simulink library "CAN_Lib_V1"  (R2018b)
settings: Solver=VariableStepAuto  StartTime=0.0  StopTime=10.0  RelTol=1e-3
undefined symbols (not defined in the file): canChannel
libraries: canmsglib x158, canlib x35, simulink x1
(part 1 of 11)
settings Model: ModifiedHistory=CAN Bus model library  Creator=E00026  LastModifiedBy=E00026
settings DataIOCC: ReturnWorkspaceOutputs=on

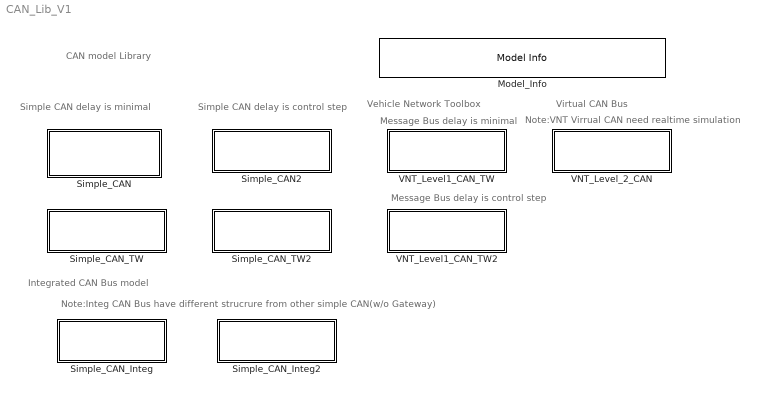
== system CAN_Lib_V1 ==
  note: Note:VNT Virrual CAN need realtime simulation
  note: Note:Integ CAN Bus have different strucrure from other simple CAN(w/o Gateway)
  note: Integrated CAN Bus model
  note: Virtual CAN Bus
  note: Message Bus delay is minimal
  note: Simple CAN delay is minimal
  note: CAN model Library
  note: Vehicle Network Toolbox
  note: Simple CAN delay is control step
  note: Message Bus delay is control step
  Model_Info : simulink/Model-Wide Utilities/Model Info  Frame=on  DisplayStringWithTags=|  HorizontalTextAlignment=Left  LeftAlignmentValue=0.02
      | Version  %<ModelVersion>
      | LastModifided by %<LastModifiedBy>  Date %<LastModificationDate>
      | Description  %<Description>
  Simple_CAN : Subsystem  VariantControl=VarObj_CanType_Simpl
  Simple_CAN2 : Subsystem  VariantControl=VarObj_CanType_Simpl
  Simple_CAN_Integ : Subsystem  VariantControl=VarObj_CanType_Simpl
  Simple_CAN_Integ2 : Subsystem  VariantControl=VarObj_CanType_Simpl
  Simple_CAN_TW : Subsystem  VariantControl=VarObj_CanType_Simpl_TW
  Simple_CAN_TW2 : Subsystem  VariantControl=VarObj_CanType_Simpl_TW
  VNT_Level1_CAN_TW : Subsystem  VariantControl=VarObj_CanType_VNT_Level_1
  VNT_Level1_CAN_TW2 : Subsystem  VariantControl=VarObj_CanType_Simpl_TW
  VNT_Level_2_CAN : Subsystem  VariantControl=VarObj_CanType_VNT_simu

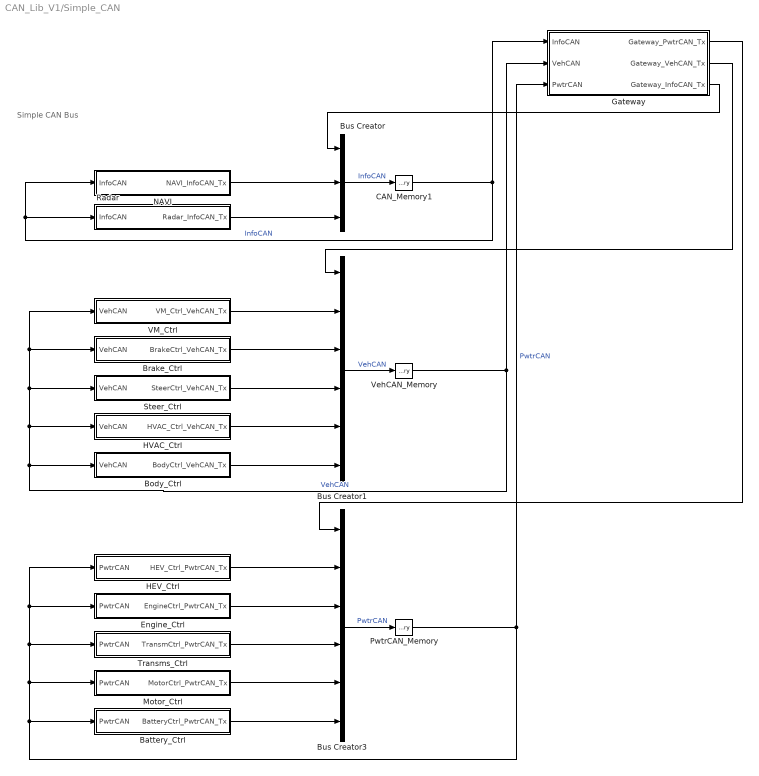
== system CAN_Lib_V1/Simple_CAN ==
  note: Simple CAN Bus
  Battery_Ctrl : Subsystem
  Body_Ctrl : Subsystem
  Brake_Ctrl : Subsystem
  Bus Creator : BusCreator  Inputs=3
  Bus Creator1 : BusCreator  Inputs=6
  Bus Creator3 : BusCreator  Inputs=6
  CAN_Memory1 : Memory
  Engine_Ctrl : Subsystem
  Gateway : Subsystem
  HEV_Ctrl : Subsystem
  HVAC_Ctrl : Subsystem
  Motor_Ctrl : Subsystem
  NAVI : Subsystem
  PwtrCAN_Memory : Memory
  Radar : Subsystem
  Steer_Ctrl : Subsystem
  Transms_Ctrl : Subsystem
  VM_Ctrl : Subsystem
  VehCAN_Memory : Memory
  wires:
  Bus Creator3/1 -> PwtrCAN_Memory/1  "PwtrCAN"
  HEV_Ctrl/1(HEV_Ctrl_PwtrCAN_Tx) -> Bus Creator3/2
  Bus Creator/1 -> CAN_Memory1/1  "InfoCAN"
  PwtrCAN_Memory/1 -> Motor_Ctrl/1(PwtrCAN), Transms_Ctrl/1(PwtrCAN), Engine_Ctrl/1(PwtrCAN), HEV_Ctrl/1(PwtrCAN), Battery_Ctrl/1(PwtrCAN), Gateway/3(PwtrCAN)  "PwtrCAN"
  Engine_Ctrl/1(EngineCtrl_PwtrCAN_Tx) -> Bus Creator3/3
  Transms_Ctrl/1(TransmCtrl_PwtrCAN_Tx) -> Bus Creator3/4
  Bus Creator1/1 -> VehCAN_Memory/1  "VehCAN"
  Battery_Ctrl/1(BatteryCtrl_PwtrCAN_Tx) -> Bus Creator3/6
  Body_Ctrl/1(BodyCtrl_VehCAN_Tx) -> Bus Creator1/6
  VehCAN_Memory/1 -> Gateway/2(VehCAN), HVAC_Ctrl/1(VehCAN), Brake_Ctrl/1(VehCAN), VM_Ctrl/1(VehCAN), Steer_Ctrl/1(VehCAN), Body_Ctrl/1(VehCAN)  "VehCAN"
  VM_Ctrl/1(VM_Ctrl_VehCAN_Tx) -> Bus Creator1/2
  Radar/1(Radar_InfoCAN_Tx) -> Bus Creator/3
  NAVI/1(NAVI_InfoCAN_Tx) -> Bus Creator/2
  Steer_Ctrl/1(SteerCtrl_VehCAN_Tx) -> Bus Creator1/4
  HVAC_Ctrl/1(HVAC_Ctrl_VehCAN_Tx) -> Bus Creator1/5
  Motor_Ctrl/1(MotorCtrl_PwtrCAN_Tx) -> Bus Creator3/5
  Brake_Ctrl/1(BrakeCtrl_VehCAN_Tx) -> Bus Creator1/3
  CAN_Memory1/1 -> Gateway/1(InfoCAN), NAVI/1(InfoCAN), Radar/1(InfoCAN)  "InfoCAN"
  Gateway/3(Gateway_InfoCAN_Tx) -> Bus Creator/1
  Gateway/2(Gateway_VehCAN_Tx) -> Bus Creator1/1
  Gateway/1(Gateway_PwtrCAN_Tx) -> Bus Creator3/1

== system CAN_Lib_V1/Simple_CAN2 ==
  note: Simple CAN Bus
  Battery_Ctrl : Subsystem
  Body_Ctrl : Subsystem
  Brake_Ctrl : Subsystem
  Bus Creator : BusCreator  Inputs=3
  Bus Creator1 : BusCreator  Inputs=6
  Bus Creator3 : BusCreator  Inputs=6
  Engine_Ctrl : Subsystem
  Gateway : Subsystem
  HEV_Ctrl : Subsystem
  HVAC_Ctrl : Subsystem
  Motor_Ctrl : Subsystem
  NAVI : Subsystem
  Radar : Subsystem
  Steer_Ctrl : Subsystem
  Transms_Ctrl : Subsystem
  VM_Ctrl : Subsystem
  wires:
  Gateway/1(Gateway_PwtrCAN_Tx) -> Bus Creator3/1
  Gateway/2(Gateway_VehCAN_Tx) -> Bus Creator1/1
  Gateway/3(Gateway_InfoCAN_Tx) -> Bus Creator/1
  Brake_Ctrl/1(BrakeCtrl_VehCAN_Tx) -> Bus Creator1/3
  Motor_Ctrl/1(MotorCtrl_PwtrCAN_Tx) -> Bus Creator3/5
  HVAC_Ctrl/1(HVAC_Ctrl_VehCAN_Tx) -> Bus Creator1/5
  Steer_Ctrl/1(SteerCtrl_VehCAN_Tx) -> Bus Creator1/4
  NAVI/1(NAVI_InfoCAN_Tx) -> Bus Creator/2
  Radar/1(Radar_InfoCAN_Tx) -> Bus Creator/3
  VM_Ctrl/1(VM_Ctrl_VehCAN_Tx) -> Bus Creator1/2
  Body_Ctrl/1(BodyCtrl_VehCAN_Tx) -> Bus Creator1/6
  Battery_Ctrl/1(BatteryCtrl_PwtrCAN_Tx) -> Bus Creator3/6
  Bus Creator1/1 -> Body_Ctrl/1(VehCAN), Steer_Ctrl/1(VehCAN), VM_Ctrl/1(VehCAN), Brake_Ctrl/1(VehCAN), HVAC_Ctrl/1(VehCAN), Gateway/2(VehCAN)  "VehCAN"
  Transms_Ctrl/1(TransmCtrl_PwtrCAN_Tx) -> Bus Creator3/4
  Engine_Ctrl/1(EngineCtrl_PwtrCAN_Tx) -> Bus Creator3/3
  Bus Creator/1 -> Radar/1(InfoCAN), NAVI/1(InfoCAN), Gateway/1(InfoCAN)  "InfoCAN"
  HEV_Ctrl/1(HEV_Ctrl_PwtrCAN_Tx) -> Bus Creator3/2
  Bus Creator3/1 -> Gateway/3(PwtrCAN), Battery_Ctrl/1(PwtrCAN), HEV_Ctrl/1(PwtrCAN), Engine_Ctrl/1(PwtrCAN), Transms_Ctrl/1(PwtrCAN), Motor_Ctrl/1(PwtrCAN)  "PwtrCAN"

== system CAN_Lib_V1/Simple_CAN_Integ ==
  note: Simple CAN Integrated Bus
  Battery_Ctrl : Subsystem
  Body_Ctrl : Subsystem
  Brake_Ctrl : Subsystem
  Bus Creator : BusCreator  Inputs=2
  Bus Creator1 : BusCreator  Inputs=5
  Bus Creator2 : BusCreator  Inputs=3
  Bus Creator3 : BusCreator  Inputs=5
  Engine_Ctrl : Subsystem
  HEV_Ctrl : Subsystem
  HVAC_Ctrl : Subsystem
  IntegCAN_Memory : Memory
  Motor_Ctrl : Subsystem
  NAVI : Subsystem
  Radar : Subsystem
  Steer_Ctrl : Subsystem
  Transms_Ctrl : Subsystem
  VM_Ctrl : Subsystem
  tag scope: CAN=scoped
  wires:
  Bus Creator2/1 -> IntegCAN_Memory/1
  IntegCAN_Memory/1 -> Battery_Ctrl/1(CAN), Motor_Ctrl/1(CAN), Transms_Ctrl/1(CAN), Engine_Ctrl/1(CAN), HEV_Ctrl/1(CAN), Body_Ctrl/1(CAN), HVAC_Ctrl/1(CAN), Steer_Ctrl/1(CAN), VM_Ctrl/1(CAN), Radar/1(CAN), NAVI/1(CAN), Brake_Ctrl/1(CAN), [CAN]  "CAN"
  Brake_Ctrl/1(BrakeCtrl_VehCAN_Tx) -> Bus Creator1/2
  Motor_Ctrl/1(MotorCtrl_PwtrCAN_Tx) -> Bus Creator3/4
  HVAC_Ctrl/1(HVAC_Ctrl_VehCAN_Tx) -> Bus Creator1/4
  Steer_Ctrl/1(SteerCtrl_VehCAN_Tx) -> Bus Creator1/3
  NAVI/1(NAVI_InfoCAN_Tx) -> Bus Creator/1
  Radar/1(Radar_InfoCAN_Tx) -> Bus Creator/2
  VM_Ctrl/1(VM_Ctrl_VehCAN_Tx) -> Bus Creator1/1
  Body_Ctrl/1(BodyCtrl_VehCAN_Tx) -> Bus Creator1/5
  Battery_Ctrl/1(BatteryCtrl_PwtrCAN_Tx) -> Bus Creator3/5
  Bus Creator1/1 -> Bus Creator2/2  "VehCAN"
  Transms_Ctrl/1(TransmCtrl_PwtrCAN_Tx) -> Bus Creator3/3
  Engine_Ctrl/1(EngineCtrl_PwtrCAN_Tx) -> Bus Creator3/2
  Bus Creator/1 -> Bus Creator2/1  "InfoCAN"
  HEV_Ctrl/1(HEV_Ctrl_PwtrCAN_Tx) -> Bus Creator3/1
  Bus Creator3/1 -> Bus Creator2/3  "PwtrCAN"

== system CAN_Lib_V1/Simple_CAN_Integ2 ==
  note: Simple CAN Integrated Bus
  Battery_Ctrl : Subsystem
  Body_Ctrl : Subsystem
  Brake_Ctrl : Subsystem
  Bus Creator : BusCreator  Inputs=2
  Bus Creator1 : BusCreator  Inputs=5
  Bus Creator2 : BusCreator  Inputs=3
  Bus Creator3 : BusCreator  Inputs=5
  Engine_Ctrl : Subsystem
  HEV_Ctrl : Subsystem
  HVAC_Ctrl : Subsystem
  Motor_Ctrl : Subsystem
  NAVI : Subsystem
  Radar : Subsystem
  Steer_Ctrl : Subsystem
  Transms_Ctrl : Subsystem
  VM_Ctrl : Subsystem
  tag scope: CAN=scoped
  wires:
  Bus Creator2/1 -> Battery_Ctrl/1(CAN), Motor_Ctrl/1(CAN), Transms_Ctrl/1(CAN), Engine_Ctrl/1(CAN), HEV_Ctrl/1(CAN), Body_Ctrl/1(CAN), HVAC_Ctrl/1(CAN), Steer_Ctrl/1(CAN), VM_Ctrl/1(CAN), Radar/1(CAN), NAVI/1(CAN), Brake_Ctrl/1(CAN), [CAN]  "CAN"
  Brake_Ctrl/1(BrakeCtrl_VehCAN_Tx) -> Bus Creator1/2
  Motor_Ctrl/1(MotorCtrl_PwtrCAN_Tx) -> Bus Creator3/4
  HVAC_Ctrl/1(HVAC_Ctrl_VehCAN_Tx) -> Bus Creator1/4
  Steer_Ctrl/1(SteerCtrl_VehCAN_Tx) -> Bus Creator1/3
  NAVI/1(NAVI_InfoCAN_Tx) -> Bus Creator/1
  Radar/1(Radar_InfoCAN_Tx) -> Bus Creator/2
  VM_Ctrl/1(VM_Ctrl_VehCAN_Tx) -> Bus Creator1/1
  Body_Ctrl/1(BodyCtrl_VehCAN_Tx) -> Bus Creator1/5
  Battery_Ctrl/1(BatteryCtrl_PwtrCAN_Tx) -> Bus Creator3/5
  Bus Creator1/1 -> Bus Creator2/2  "VehCAN"
  Transms_Ctrl/1(TransmCtrl_PwtrCAN_Tx) -> Bus Creator3/3
  Engine_Ctrl/1(EngineCtrl_PwtrCAN_Tx) -> Bus Creator3/2
  Bus Creator/1 -> Bus Creator2/1  "InfoCAN"
  HEV_Ctrl/1(HEV_Ctrl_PwtrCAN_Tx) -> Bus Creator3/1
  Bus Creator3/1 -> Bus Creator2/3  "PwtrCAN"

== system CAN_Lib_V1/Simple_CAN_TW ==
  note: Simple CAN Bus
  Battery_Ctrl : Subsystem
  Body_Ctrl : Subsystem
  Brake_Ctrl : Subsystem
  Engine_Ctrl : Subsystem
  Gateway : Subsystem
  HEV_Ctrl : Subsystem
  HVAC_Ctrl : Subsystem
  InfoCAN : Subsystem
  Motor_Ctrl : Subsystem
  NAVI : Subsystem
  PwtrCAN : Subsystem
  Radar : Subsystem
  Steer_Ctrl : Subsystem
  Transms_Ctrl : Subsystem
  VM_Ctrl : Subsystem
  VehCAN : Subsystem
  connections:
  InfoCAN/LConn1 -- NAVI/RConn1
  InfoCAN/LConn2 -- Radar/RConn1
  Gateway/LConn1 -- InfoCAN/RConn1
  VehCAN/RConn1 -- Gateway/LConn2
  Gateway/RConn1 -- PwtrCAN/LConn1
  VM_Ctrl/RConn1 -- VehCAN/LConn1
  Brake_Ctrl/RConn1 -- VehCAN/LConn2
  Steer_Ctrl/RConn1 -- VehCAN/LConn3
  HVAC_Ctrl/RConn1 -- VehCAN/LConn4
  Body_Ctrl/RConn1 -- VehCAN/LConn5
  PwtrCAN/RConn1 -- HEV_Ctrl/LConn1
  PwtrCAN/RConn2 -- Engine_Ctrl/LConn1
  PwtrCAN/RConn3 -- Transms_Ctrl/LConn1
  PwtrCAN/RConn4 -- Motor_Ctrl/LConn1
  PwtrCAN/RConn5 -- Battery_Ctrl/LConn1

== system CAN_Lib_V1/Simple_CAN_TW2 ==
  note: Simple CAN Bus
  Battery_Ctrl : Subsystem
  Body_Ctrl : Subsystem
  Brake_Ctrl : Subsystem
  Engine_Ctrl : Subsystem
  Gateway : Subsystem
  HEV_Ctrl : Subsystem
  HVAC_Ctrl : Subsystem
  InfoCAN : Subsystem
  Motor_Ctrl : Subsystem
  NAVI : Subsystem
  PwtrCAN : Subsystem
  Radar : Subsystem
  Steer_Ctrl : Subsystem
  Transms_Ctrl : Subsystem
  VM_Ctrl : Subsystem
  VehCAN : Subsystem
  connections:
  PwtrCAN/RConn5 -- Battery_Ctrl/LConn1
  PwtrCAN/RConn4 -- Motor_Ctrl/LConn1
  PwtrCAN/RConn3 -- Transms_Ctrl/LConn1
  PwtrCAN/RConn2 -- Engine_Ctrl/LConn1
  PwtrCAN/RConn1 -- HEV_Ctrl/LConn1
  Body_Ctrl/RConn1 -- VehCAN/LConn5
  HVAC_Ctrl/RConn1 -- VehCAN/LConn4
  Steer_Ctrl/RConn1 -- VehCAN/LConn3
  Brake_Ctrl/RConn1 -- VehCAN/LConn2
  VM_Ctrl/RConn1 -- VehCAN/LConn1
  Gateway/RConn1 -- PwtrCAN/LConn1
  VehCAN/RConn1 -- Gateway/LConn2
  Gateway/LConn1 -- InfoCAN/RConn1
  InfoCAN/LConn2 -- Radar/RConn1
  InfoCAN/LConn1 -- NAVI/RConn1

== system CAN_Lib_V1/VNT_Level1_CAN_TW ==
  note: VNT Level1 CAN Bus
  Battery_Ctrl : Subsystem
  Body_Ctrl : Subsystem
  Brake_Ctrl : Subsystem
  Engine_Ctrl : Subsystem
  Gateway : Subsystem
  HEV_Ctrl : Subsystem
  HVAC_Ctrl : Subsystem
  InfoCAN : Subsystem
  Motor_Ctrl : Subsystem
  NAVI : Subsystem
  PwtrCAN : Subsystem
  Radar : Subsystem
  Steer_Ctrl : Subsystem
  Transms_Ctrl : Subsystem
  VM_Ctrl : Subsystem
  VehCAN : Subsystem
  connections:
  InfoCAN/LConn1 -- NAVI/RConn1
  InfoCAN/LConn2 -- Radar/RConn1
  Gateway/LConn1 -- InfoCAN/RConn1
  VehCAN/RConn1 -- Gateway/LConn2
  Gateway/RConn1 -- PwtrCAN/LConn1
  VM_Ctrl/RConn1 -- VehCAN/LConn1
  Brake_Ctrl/RConn1 -- VehCAN/LConn2
  Steer_Ctrl/RConn1 -- VehCAN/LConn3
  HVAC_Ctrl/RConn1 -- VehCAN/LConn4
  Body_Ctrl/RConn1 -- VehCAN/LConn5
  PwtrCAN/RConn1 -- HEV_Ctrl/LConn1
  PwtrCAN/RConn2 -- Engine_Ctrl/LConn1
  PwtrCAN/RConn3 -- Transms_Ctrl/LConn1
  PwtrCAN/RConn4 -- Motor_Ctrl/LConn1
  PwtrCAN/RConn5 -- Battery_Ctrl/LConn1

== system CAN_Lib_V1/VNT_Level1_CAN_TW2 ==
  note: VNT Level1 CAN Bus
  Battery_Ctrl : Subsystem
  Body_Ctrl : Subsystem
  Brake_Ctrl : Subsystem
  Engine_Ctrl : Subsystem
  Gateway : Subsystem
  HEV_Ctrl : Subsystem
  HVAC_Ctrl : Subsystem
  InfoCAN : Subsystem
  Motor_Ctrl : Subsystem
  NAVI : Subsystem
  PwtrCAN : Subsystem
  Radar : Subsystem
  Steer_Ctrl : Subsystem
  Transms_Ctrl : Subsystem
  VM_Ctrl : Subsystem
  VehCAN : Subsystem
  connections:
  PwtrCAN/RConn5 -- Battery_Ctrl/LConn1
  PwtrCAN/RConn4 -- Motor_Ctrl/LConn1
  PwtrCAN/RConn3 -- Transms_Ctrl/LConn1
  PwtrCAN/RConn2 -- Engine_Ctrl/LConn1
  PwtrCAN/RConn1 -- HEV_Ctrl/LConn1
  Body_Ctrl/RConn1 -- VehCAN/LConn5
  HVAC_Ctrl/RConn1 -- VehCAN/LConn4
  Steer_Ctrl/RConn1 -- VehCAN/LConn3
  Brake_Ctrl/RConn1 -- VehCAN/LConn2
  VM_Ctrl/RConn1 -- VehCAN/LConn1
  Gateway/RConn1 -- PwtrCAN/LConn1
  VehCAN/RConn1 -- Gateway/LConn2
  Gateway/LConn1 -- InfoCAN/RConn1
  InfoCAN/LConn2 -- Radar/RConn1
  InfoCAN/LConn1 -- NAVI/RConn1

== system CAN_Lib_V1/VNT_Level_2_CAN ==
  note: VNT Level_2 CAN Bus
  Battery_Ctrl : Subsystem
  Body_Ctrl : Subsystem
  Brake_Ctrl : Subsystem
  CAN Configuration : canlib/CAN Configuration  BlockHandle=36204.0016  DeviceMenu=MathWorks Virtual 1 (Channel 1)  Device=MathWorks Virtual 1 (Channel 1)  ObjConstructor=canChannel('MathWorks','Virtual 1',1)  BusSpeed=500000  EnableBitParameters=off  AckMode=Normal
      settings: SourceProductName=Vehicle Network Toolbox  SourceProductBaseCode=VN
  CAN Configuration1 : canlib/CAN Configuration  BlockHandle=36205.0016  DeviceMenu=MathWorks Virtual 1 (Channel 2)  Device=MathWorks Virtual 1 (Channel 2)  ObjConstructor=canChannel('MathWorks','Virtual 1',2)  BusSpeed=500000  EnableBitParameters=off  AckMode=Normal
      settings: SourceProductName=Vehicle Network Toolbox  SourceProductBaseCode=VN
  Engine_Ctrl : Subsystem
  Gateway : Subsystem
  HEV_Ctrl : Subsystem
  HVAC_Ctrl : Subsystem
  Motor_Ctrl : Subsystem
  NAVI : Subsystem
  Radar : Subsystem
  Steer_Ctrl : Subsystem
  Transms_Ctrl : Subsystem
  VM_Ctrl : Subsystem

== system CAN_Lib_V1/Simple_CAN/Battery_Ctrl ==
  note: Battery control
  note: CAN receive and transmit
  note: Battery Control
  PwtrCAN : Inport
  Bus Creator5 : BusCreator  Inputs=1
  Bus Selector : BusSelector  OutputSignals=HEV_Ctrl_PwtrCAN_Tx.HEVCtrl_Motor_torque_request
  Rate Transition1 : RateTransition  Deterministic=off
      settings: AttributesFormatString=<Deterministic=%<Deterministic>>
  Rate Transition2 : RateTransition  Deterministic=off
      settings: AttributesFormatString=<Deterministic=%<Deterministic>>
  BatteryCtrl_PwtrCAN_Tx : Outport
  tag scope: BatteryCtrl_PwtrCAN_Rx=scoped
  wires:
  Bus Selector/1 -> Bus Creator5/1  "<HEVCtrl_Motor_torque_request>"
  PwtrCAN/1 -> Bus Selector/1
  Bus Creator5/1 -> Rate Transition1/1
  [BatteryCtrl_PwtrCAN_Tx] -> Rate Transition2/1
  Rate Transition1/1 -> [BatteryCtrl_PwtrCAN_Rx]  "BatteryCtrl_PwtrCAN_Rx"
  Rate Transition2/1 -> BatteryCtrl_PwtrCAN_Tx/1  "BatteryCtrl_PwtrCAN_Tx"

== system CAN_Lib_V1/Simple_CAN/Body_Ctrl ==
  note: Body control
  note: CAN receive and transmit
  note: Body Control
  VehCAN : Inport
  Bus Creator : BusCreator  Inputs=3
  Bus Selector3 : BusSelector  OutputSignals=BrakeCtrl_VehCAN_Tx.BrkCtrl_Vehicle_speed,Gateway_VehCAN_Tx.EngCtrl_Engine_speed,Gateway_VehCAN_Tx.HEVCtrl_IdleStop_status
  Rate Transition1 : RateTransition  Deterministic=off
      settings: AttributesFormatString=<Deterministic=%<Deterministic>>
  Rate Transition2 : RateTransition  Deterministic=off
      settings: AttributesFormatString=<Deterministic=%<Deterministic>>
  BodyCtrl_VehCAN_Tx : Outport
  tag scope: BodyCtrl_VehCAN_Rx=scoped
  wires:
  Bus Creator/1 -> Rate Transition1/1
  Bus Selector3/1 -> Bus Creator/1  "<BrkCtrl_Vehicle_speed>"
  Bus Selector3/2 -> Bus Creator/2  "<EngCtrl_Engine_speed>"
  VehCAN/1 -> Bus Selector3/1
  [BodyCtrl_VehCAN_Tx] -> Rate Transition2/1
  Rate Transition1/1 -> [BodyCtrl_VehCAN_Rx]  "BodyCtrl_VehCAN_Rx"
  Rate Transition2/1 -> BodyCtrl_VehCAN_Tx/1  "BodyCtrl_VehCAN_Tx"
  Bus Selector3/3 -> Bus Creator/3  "<HEVCtrl_IdleStop_status>"

== system CAN_Lib_V1/Simple_CAN/Brake_Ctrl ==
  note: Brake control
  note: CAN receive and transmit
  note: Brake Control
  VehCAN : Inport
  Bus Creator : BusCreator  Inputs=4
  Bus Selector3 : BusSelector  OutputSignals=Gateway_VehCAN_Tx.HEVCtrl_Regen_brake_torque_available,Gateway_VehCAN_Tx.HEVCtrl_Regen_brake_torque_actual,VM_Ctrl_VehCAN_Tx.VMCtrl_BrakeForceStatus,VM_Ctrl_VehCAN_Tx.VMCtrl_BrakeForceCmnd
  Rate Transition1 : RateTransition  Deterministic=off
      settings: AttributesFormatString=<Deterministic=%<Deterministic>>
  Rate Transition2 : RateTransition  Deterministic=off
      settings: AttributesFormatString=<Deterministic=%<Deterministic>>
  BrakeCtrl_VehCAN_Tx : Outport
  tag scope: BrakeCtrl_VehCAN_Rx=scoped
  wires:
  Bus Creator/1 -> Rate Transition1/1
  Bus Selector3/2 -> Bus Creator/2  "<HEVCtrl_Regen_brake_torque_actual>"
  Bus Selector3/1 -> Bus Creator/1  "<HEVCtrl_Regen_brake_torque_available>"
  VehCAN/1 -> Bus Selector3/1
  [BrakeCtrl_VehCAN_Tx] -> Rate Transition2/1
  Rate Transition1/1 -> [BrakeCtrl_VehCAN_Rx]  "BrakeCtrl_VehCAN_Rx"
  Rate Transition2/1 -> BrakeCtrl_VehCAN_Tx/1  "BrakeCtrl_VehCAN_Tx"
  Bus Selector3/3 -> Bus Creator/3  "<VMCtrl_BrakeForceStatus>"
  Bus Selector3/4 -> Bus Creator/4  "<VMCtrl_BrakeForceCmnd>"

== system CAN_Lib_V1/Simple_CAN/Engine_Ctrl ==
  note: Engine control
  note: Engine Control
  note: CAN receive and transmit
  PwtrCAN : Inport
  Bus Creator5 : BusCreator  Inputs=4
  Bus Selector : BusSelector  OutputSignals=HEV_Ctrl_PwtrCAN_Tx.HEVCtrl_Engine_torque_request,HEV_Ctrl_PwtrCAN_Tx.HEVCtrl_IdleStop_preparation_request,HEV_Ctrl_PwtrCAN_Tx.HEVCtrl_IdleStop_request,HEV_Ctrl_PwtrCAN_Tx.HEVCtrl_IdleStop_status
  Rate Transition1 : RateTransition  Deterministic=off
      settings: AttributesFormatString=<Deterministic=%<Deterministic>>
  Rate Transition2 : RateTransition  Deterministic=off
      settings: AttributesFormatString=<Deterministic=%<Deterministic>>
  EngineCtrl_PwtrCAN_Tx : Outport
  tag scope: EngineCtrl_PwtrCAN_Rx=scoped
  wires:
  [EngineCtrl_PwtrCAN_Tx] -> Rate Transition2/1
  PwtrCAN/1 -> Bus Selector/1
  Bus Creator5/1 -> Rate Transition1/1
  Bus Selector/1 -> Bus Creator5/1  "<HEVCtrl_Engine_torque_request>"
  Rate Transition1/1 -> [EngineCtrl_PwtrCAN_Rx]  "EngineCtrl_PwtrCAN_Rx"
  Rate Transition2/1 -> EngineCtrl_PwtrCAN_Tx/1  "EngineCtrl_PwtrCAN_Tx"
  Bus Selector/2 -> Bus Creator5/2  "<HEVCtrl_IdleStop_preparation_request>"
  Bus Selector/3 -> Bus Creator5/3  "<HEVCtrl_IdleStop_request>"
  Bus Selector/4 -> Bus Creator5/4  "<HEVCtrl_IdleStop_status>"

== system CAN_Lib_V1/Simple_CAN/Gateway ==
  note: Gateway
  InfoCAN : Inport
  VehCAN : Inport  Port=2
  PwtrCAN : Inport  Port=3
  Gateway_InfoCAN : Subsystem
  Gateway_PwtrCAN : Subsystem
  Gateway_VehCAN : Subsystem
  Info Hub : Subsystem
  Gateway_PwtrCAN_Tx : Outport
  Gateway_VehCAN_Tx : Outport  Port=2
  Gateway_InfoCAN_Tx : Outport  Port=3
  wires:
  InfoCAN/1 -> Info Hub/1(InfoCAN), Gateway_PwtrCAN/1(InfoCAN), Gateway_VehCAN/1(InfoCAN)
  PwtrCAN/1 -> Info Hub/3(PwtrCAN), Gateway_VehCAN/2(PwtrCAN)
  VehCAN/1 -> Gateway_InfoCAN/1(VehCAN), Info Hub/2(VehCAN), Gateway_PwtrCAN/2(VehCAN)
  Gateway_InfoCAN/1(Gateway_InfoCAN_Tx) -> Gateway_InfoCAN_Tx/1
  Gateway_VehCAN/1(Gateway_VehCAN_Tx) -> Gateway_VehCAN_Tx/1
  Gateway_PwtrCAN/1(Gateway_PwtrCAN_Tx) -> Gateway_PwtrCAN_Tx/1

== system CAN_Lib_V1/Simple_CAN/HEV_Ctrl ==
  note: HEV control
  note: HEV control
  note: CAN receive and transmit
  PwtrCAN : Inport
  Bus Creator1 : BusCreator  Inputs=13
  Bus Selector3 : BusSelector  OutputSignals=BatteryCtrl_PwtrCAN_Tx.BatCtrl_SOC,TransmCtrl_PwtrCAN_Tx.TmCtrl_Clutch_position,TransmCtrl_PwtrCAN_Tx.TmCtrl_Gear_position,Gateway_PwtrCAN_Tx.BrkCtrl_Vehicle_speed,Gateway_PwtrCAN_Tx.BrkCtrl_Regen_brake_torque_request,MotorCtrl_PwtrCAN_Tx.MtrCtrl_Motor_torque_actual,MotorCtrl_PwtrCAN_Tx.MtrCtrl_Motor_torque_available,MotorCtrl_PwtrCAN_Tx.MtrCtrl_Motor_regen_torque_available,EngineCtrl_PwtrCAN_Tx.EngCtrl_Engine_speed,EngineCtrl_PwtrCAN_Tx.EngCtrl_Engine_torque_actual,Gateway_PwtrCAN_Tx.VMCtrl_PropTorqStatus,Gateway_PwtrCAN_Tx.VMCtrl_PropTorqCmnd,Gateway_PwtrCAN_Tx.NAVI_Home_around_status
  Rate Transition1 : RateTransition  Deterministic=off
      settings: AttributesFormatString=<Deterministic=%<Deterministic>>
  Rate Transition4 : RateTransition  Deterministic=off
      settings: AttributesFormatString=<Deterministic=%<Deterministic>>
  HEV_Ctrl_PwtrCAN_Tx : Outport
  tag scope: HEV_Ctrl_PwtrCAN_Rx=scoped
  wires:
  Bus Creator1/1 -> Rate Transition1/1
  Bus Selector3/10 -> Bus Creator1/10  "<EngCtrl_Engine_torque_actual>"
  Bus Selector3/9 -> Bus Creator1/9  "<EngCtrl_Engine_speed>"
  Bus Selector3/8 -> Bus Creator1/8  "<MtrCtrl_Motor_regen_torque_available>"
  Bus Selector3/7 -> Bus Creator1/7  "<MtrCtrl_Motor_torque_available>"
  Bus Selector3/6 -> Bus Creator1/6  "<MtrCtrl_Motor_torque_actual>"
  Bus Selector3/5 -> Bus Creator1/5  "<BrkCtrl_Regen_brake_torque_request>"
  Bus Selector3/4 -> Bus Creator1/4  "<BrkCtrl_Vehicle_speed>"
  Bus Selector3/3 -> Bus Creator1/3  "<TmCtrl_Gear_position>"
  Bus Selector3/2 -> Bus Creator1/2  "<TmCtrl_Clutch_position>"
  Bus Selector3/1 -> Bus Creator1/1  "<BatCtrl_SOC>"
  PwtrCAN/1 -> Bus Selector3/1
  [HEV_Ctrl_PwtrCAN_Tx] -> Rate Transition4/1
  Rate Transition4/1 -> HEV_Ctrl_PwtrCAN_Tx/1  "HEV_Ctrl_PwtrCAN_Tx"
  Rate Transition1/1 -> [HEV_Ctrl_PwtrCAN_Rx]  "HEV_Ctrl_PwtrCAN_Rx"
  Bus Selector3/11 -> Bus Creator1/11  "<VMCtrl_PropTorqStatus>"
  Bus Selector3/12 -> Bus Creator1/12  "<VMCtrl_PropTorqCmnd>"
  Bus Selector3/13 -> Bus Creator1/13  "<NAVI_Home_around_status>"

== system CAN_Lib_V1/Simple_CAN/HVAC_Ctrl ==
  note: HVAC control
  note: CAN receive and transmit
  note: HVAC Control
  VehCAN : Inport
  Bus Creator : BusCreator  Inputs=3
  Bus Selector : BusSelector  OutputSignals=Gateway_VehCAN_Tx.EngCtrl_Engine_speed,Gateway_VehCAN_Tx.HEVCtrl_IdleStop_preparation_request,Gateway_VehCAN_Tx.HEVCtrl_IdleStop_status
  Rate Transition1 : RateTransition  Deterministic=off
      settings: AttributesFormatString=<Deterministic=%<Deterministic>>
  Rate Transition2 : RateTransition  Deterministic=off
      settings: AttributesFormatString=<Deterministic=%<Deterministic>>
  HVAC_Ctrl_VehCAN_Tx : Outport
  tag scope: HVAC_Ctrl_VehCAN_Rx=scoped
  wires:
  Bus Creator/1 -> Rate Transition1/1
  Bus Selector/1 -> Bus Creator/1  "<EngCtrl_Engine_speed>"
  VehCAN/1 -> Bus Selector/1
  [HVAC_Ctrl_VehCAN_Tx] -> Rate Transition2/1
  Rate Transition1/1 -> [HVAC_Ctrl_VehCAN_Rx]  "HVAC_Ctrl_VehCAN_Rx"
  Rate Transition2/1 -> HVAC_Ctrl_VehCAN_Tx/1  "HVAC_Ctrl_VehCAN_Tx"
  Bus Selector/2 -> Bus Creator/2  "<HEVCtrl_IdleStop_preparation_request>"
  Bus Selector/3 -> Bus Creator/3  "<HEVCtrl_IdleStop_status>"

== system CAN_Lib_V1/Simple_CAN/Motor_Ctrl ==
  note: Motor control
  note: Motor Control
  note: CAN receive and transmit
  PwtrCAN : Inport
  Bus Creator7 : BusCreator  Inputs=3
  Bus Selector2 : BusSelector  OutputSignals=TransmCtrl_PwtrCAN_Tx.TmCtrl_Clutch_position,HEV_Ctrl_PwtrCAN_Tx.HEVCtrl_Motor_torque_request,EngineCtrl_PwtrCAN_Tx.EngCtrl_Engine_speed
  Rate Transition1 : RateTransition  Deterministic=off
      settings: AttributesFormatString=<Deterministic=%<Deterministic>>
  Rate Transition2 : RateTransition  Deterministic=off
      settings: AttributesFormatString=<Deterministic=%<Deterministic>>
  MotorCtrl_PwtrCAN_Tx : Outport
  tag scope: MotorCtrl_PwtrCAN_Rx=scoped
  wires:
  [MotorCtrl_PwtrCAN_Tx] -> Rate Transition2/1
  Rate Transition1/1 -> [MotorCtrl_PwtrCAN_Rx]  "MotorCtrl_PwtrCAN_Rx"
  Bus Selector2/2 -> Bus Creator7/2  "<HEVCtrl_Motor_torque_request>"
  Bus Creator7/1 -> Rate Transition1/1
  Bus Selector2/3 -> Bus Creator7/3  "<EngCtrl_Engine_speed>"
  Bus Selector2/1 -> Bus Creator7/1  "<TmCtrl_Clutch_position>"
  Rate Transition2/1 -> MotorCtrl_PwtrCAN_Tx/1  "MotorCtrl_PwtrCAN_Tx"
  PwtrCAN/1 -> Bus Selector2/1

== system CAN_Lib_V1/Simple_CAN/NAVI ==
  note: Navigation
  note: CAN receive and transmit
  note: Navigation
  InfoCAN : Inport
  Bus Creator : BusCreator  Inputs=1
  Bus Selector1 : BusSelector  OutputSignals=Gateway_InfoCAN_Tx.BrkCtrl_Vehicle_speed
  Rate Transition1 : RateTransition  Deterministic=off
      settings: AttributesFormatString=<Deterministic=%<Deterministic>>
  Rate Transition2 : RateTransition  Deterministic=off
      settings: AttributesFormatString=<Deterministic=%<Deterministic>>
  NAVI_InfoCAN_Tx : Outport
  tag scope: NAVI_InfoCAN_Rx=scoped
  wires:
  Bus Creator/1 -> Rate Transition1/1
  Bus Selector1/1 -> Bus Creator/1  "<BrkCtrl_Vehicle_speed>"
  InfoCAN/1 -> Bus Selector1/1
  [NAVI_InfoCAN_Tx] -> Rate Transition2/1
  Rate Transition1/1 -> [NAVI_InfoCAN_Rx]  "NAVI_InfoCAN_Rx"
  Rate Transition2/1 -> NAVI_InfoCAN_Tx/1  "NAVI_InfoCAN_Tx"

== system CAN_Lib_V1/Simple_CAN/Radar ==
  note: Radar detection
  note: CAN receive and transmit
  note: Radar Detection
  InfoCAN : Inport
  Bus Creator : BusCreator  Inputs=1
  Bus Selector1 : BusSelector  OutputSignals=Gateway_InfoCAN_Tx.BrkCtrl_Vehicle_speed
  Rate Transition1 : RateTransition  Deterministic=off
      settings: AttributesFormatString=<Deterministic=%<Deterministic>>
  Rate Transition2 : RateTransition  Deterministic=off
      settings: AttributesFormatString=<Deterministic=%<Deterministic>>
  Radar_InfoCAN_Tx : Outport
  tag scope: Radar_InfoCAN_Rx=scoped
  wires:
  InfoCAN/1 -> Bus Selector1/1
  Bus Creator/1 -> Rate Transition1/1
  Bus Selector1/1 -> Bus Creator/1  "<BrkCtrl_Vehicle_speed>"
  [Radar_InfoCAN_Tx] -> Rate Transition2/1
  Rate Transition1/1 -> [Radar_InfoCAN_Rx]  "Radar_InfoCAN_Rx"
  Rate Transition2/1 -> Radar_InfoCAN_Tx/1  "Radar_InfoCAN_Tx"

== system CAN_Lib_V1/Simple_CAN/Steer_Ctrl ==
  note: Steering control
  note: CAN receive and transmit
  note: Steering Control
  VehCAN : Inport
  Bus Creator : BusCreator  Inputs=1
  Bus Selector1 : BusSelector  OutputSignals=BrakeCtrl_VehCAN_Tx.BrkCtrl_Vehicle_speed
  Rate Transition1 : RateTransition  Deterministic=off
      settings: AttributesFormatString=<Deterministic=%<Deterministic>>
  Rate Transition2 : RateTransition  Deterministic=off
      settings: AttributesFormatString=<Deterministic=%<Deterministic>>
  SteerCtrl_VehCAN_Tx : Outport
  tag scope: SteerCtrl_VehCAN_Rx=scoped
  wires:
  Bus Creator/1 -> Rate Transition1/1
  Bus Selector1/1 -> Bus Creator/1  "<BrkCtrl_Vehicle_speed>"
  VehCAN/1 -> Bus Selector1/1
  [SteerCtrl_VehCAN_Tx] -> Rate Transition2/1
  Rate Transition1/1 -> [SteerCtrl_VehCAN_Rx]  "SteerCtrl_VehCAN_Rx"
  Rate Transition2/1 -> SteerCtrl_VehCAN_Tx/1  "SteerCtrl_VehCAN_Tx"

== system CAN_Lib_V1/Simple_CAN/Transms_Ctrl ==
  note: Transmission control
  note: CAN receive and transmit
  note: Transmission Control
  PwtrCAN : Inport
  Bus Creator6 : BusCreator  Inputs=2
  Bus Selector1 : BusSelector  OutputSignals=Gateway_PwtrCAN_Tx.BrkCtrl_Vehicle_speed,EngineCtrl_PwtrCAN_Tx.EngCtrl_Engine_speed
  Rate Transition1 : RateTransition  Deterministic=off
      settings: AttributesFormatString=<Deterministic=%<Deterministic>>
  Rate Transition2 : RateTransition  Deterministic=off
      settings: AttributesFormatString=<Deterministic=%<Deterministic>>
  TransmCtrl_PwtrCAN_Tx : Outport
  tag scope: TransmCtrl_PwtrCAN_Rx=scoped
  wires:
  [TransmCtrl_PwtrCAN_Tx] -> Rate Transition2/1
  Rate Transition2/1 -> TransmCtrl_PwtrCAN_Tx/1  "TransmCtrl_PwtrCAN_Tx"
  Bus Creator6/1 -> Rate Transition1/1
  Bus Selector1/2 -> Bus Creator6/2  "<EngCtrl_Engine_speed>"
  Bus Selector1/1 -> Bus Creator6/1  "<BrkCtrl_Vehicle_speed>"
  PwtrCAN/1 -> Bus Selector1/1
  Rate Transition1/1 -> [TransmCtrl_PwtrCAN_Rx]  "TransmCtrl_PwtrCAN_Rx"

== system CAN_Lib_V1/Simple_CAN/VM_Ctrl ==
  note: Vehicle motion control
  note: Vehicle Motion Control
  note: CAN receive and transmit
  VehCAN : Inport
  Bus Creator : BusCreator  Inputs=1
  Bus Selector1 : BusSelector  OutputSignals=BrakeCtrl_VehCAN_Tx.BrkCtrl_Vehicle_speed
  Rate Transition1 : RateTransition  Deterministic=off
      settings: AttributesFormatString=<Deterministic=%<Deterministic>>
  Rate Transition2 : RateTransition  Deterministic=off
      settings: AttributesFormatString=<Deterministic=%<Deterministic>>
  VM_Ctrl_VehCAN_Tx : Outport
  tag scope: VM_Ctrl_VehCAN_Rx=scoped
  wires:
  Bus Creator/1 -> Rate Transition1/1
  Bus Selector1/1 -> Bus Creator/1  "<BrkCtrl_Vehicle_speed>"
  VehCAN/1 -> Bus Selector1/1
  [VM_Ctrl_VehCAN_Tx] -> Rate Transition2/1
  Rate Transition1/1 -> [VM_Ctrl_VehCAN_Rx]  "VM_Ctrl_VehCAN_Rx"
  Rate Transition2/1 -> VM_Ctrl_VehCAN_Tx/1  "VM_Ctrl_VehCAN_Tx"

== system CAN_Lib_V1/Simple_CAN2/Battery_Ctrl ==
  note: Battery Control
  note: CAN receive and transmit
  note: Battery control
  PwtrCAN : Inport
  Bus Creator5 : BusCreator  Inputs=1
  Bus Selector : BusSelector  OutputSignals=HEV_Ctrl_PwtrCAN_Tx.HEVCtrl_Motor_torque_request
  Rate Transition1 : RateTransition  Deterministic=off
      settings: AttributesFormatString=<Deterministic=%<Deterministic>>
  Unit Delay : UnitDelay  SampleTime=-1
  BatteryCtrl_PwtrCAN_Tx : Outport
  tag scope: BatteryCtrl_PwtrCAN_Rx=scoped
  wires:
  Unit Delay/1 -> BatteryCtrl_PwtrCAN_Tx/1  "BatteryCtrl_PwtrCAN_Tx"
  Rate Transition1/1 -> [BatteryCtrl_PwtrCAN_Rx]  "BatteryCtrl_PwtrCAN_Rx"
  [BatteryCtrl_PwtrCAN_Tx] -> Unit Delay/1
  Bus Creator5/1 -> Rate Transition1/1
  PwtrCAN/1 -> Bus Selector/1
  Bus Selector/1 -> Bus Creator5/1  "<HEVCtrl_Motor_torque_request>"

== system CAN_Lib_V1/Simple_CAN2/Body_Ctrl ==
  note: Body Control
  note: CAN receive and transmit
  note: Body control
  VehCAN : Inport
  Bus Creator : BusCreator  Inputs=3
  Bus Selector3 : BusSelector  OutputSignals=BrakeCtrl_VehCAN_Tx.BrkCtrl_Vehicle_speed,Gateway_VehCAN_Tx.EngCtrl_Engine_speed,Gateway_VehCAN_Tx.HEVCtrl_IdleStop_status
  Rate Transition1 : RateTransition  Deterministic=off
      settings: AttributesFormatString=<Deterministic=%<Deterministic>>
  Unit Delay : UnitDelay  SampleTime=-1
  BodyCtrl_VehCAN_Tx : Outport
  tag scope: BodyCtrl_VehCAN_Rx=scoped
  wires:
  Bus Selector3/3 -> Bus Creator/3  "<HEVCtrl_IdleStop_status>"
  Unit Delay/1 -> BodyCtrl_VehCAN_Tx/1  "BodyCtrl_VehCAN_Tx"
  Rate Transition1/1 -> [BodyCtrl_VehCAN_Rx]  "BodyCtrl_VehCAN_Rx"
  [BodyCtrl_VehCAN_Tx] -> Unit Delay/1
  VehCAN/1 -> Bus Selector3/1
  Bus Selector3/2 -> Bus Creator/2  "<EngCtrl_Engine_speed>"
  Bus Selector3/1 -> Bus Creator/1  "<BrkCtrl_Vehicle_speed>"
  Bus Creator/1 -> Rate Transition1/1

== system CAN_Lib_V1/Simple_CAN2/Brake_Ctrl ==
  note: Brake Control
  note: CAN receive and transmit
  note: Brake control
  VehCAN : Inport
  Bus Creator : BusCreator  Inputs=4
  Bus Selector3 : BusSelector  OutputSignals=Gateway_VehCAN_Tx.HEVCtrl_Regen_brake_torque_available,Gateway_VehCAN_Tx.HEVCtrl_Regen_brake_torque_actual,VM_Ctrl_VehCAN_Tx.VMCtrl_BrakeForceStatus,VM_Ctrl_VehCAN_Tx.VMCtrl_BrakeForceCmnd
  Rate Transition1 : RateTransition  Deterministic=off
      settings: AttributesFormatString=<Deterministic=%<Deterministic>>
  Unit Delay : UnitDelay  SampleTime=-1
  BrakeCtrl_VehCAN_Tx : Outport
  tag scope: BrakeCtrl_VehCAN_Rx=scoped
  wires:
  Bus Selector3/4 -> Bus Creator/4  "<VMCtrl_BrakeForceCmnd>"
  Bus Selector3/3 -> Bus Creator/3  "<VMCtrl_BrakeForceStatus>"
  Unit Delay/1 -> BrakeCtrl_VehCAN_Tx/1  "BrakeCtrl_VehCAN_Tx"
  Rate Transition1/1 -> [BrakeCtrl_VehCAN_Rx]  "BrakeCtrl_VehCAN_Rx"
  [BrakeCtrl_VehCAN_Tx] -> Unit Delay/1
  VehCAN/1 -> Bus Selector3/1
  Bus Selector3/1 -> Bus Creator/1  "<HEVCtrl_Regen_brake_torque_available>"
  Bus Selector3/2 -> Bus Creator/2  "<HEVCtrl_Regen_brake_torque_actual>"
  Bus Creator/1 -> Rate Transition1/1

== system CAN_Lib_V1/Simple_CAN2/Engine_Ctrl ==
  note: CAN receive and transmit
  note: Engine Control
  note: Engine control
  PwtrCAN : Inport
  Bus Creator5 : BusCreator  Inputs=4
  Bus Selector : BusSelector  OutputSignals=HEV_Ctrl_PwtrCAN_Tx.HEVCtrl_Engine_torque_request,HEV_Ctrl_PwtrCAN_Tx.HEVCtrl_IdleStop_preparation_request,HEV_Ctrl_PwtrCAN_Tx.HEVCtrl_IdleStop_request,HEV_Ctrl_PwtrCAN_Tx.HEVCtrl_IdleStop_status
  Rate Transition1 : RateTransition  Deterministic=off
      settings: AttributesFormatString=<Deterministic=%<Deterministic>>
  Unit Delay : UnitDelay  SampleTime=-1
  EngineCtrl_PwtrCAN_Tx : Outport
  tag scope: EngineCtrl_PwtrCAN_Rx=scoped
  wires:
  Bus Selector/4 -> Bus Creator5/4  "<HEVCtrl_IdleStop_status>"
  Bus Selector/3 -> Bus Creator5/3  "<HEVCtrl_IdleStop_request>"
  Bus Selector/2 -> Bus Creator5/2  "<HEVCtrl_IdleStop_preparation_request>"
  Unit Delay/1 -> EngineCtrl_PwtrCAN_Tx/1  "EngineCtrl_PwtrCAN_Tx"
  Rate Transition1/1 -> [EngineCtrl_PwtrCAN_Rx]  "EngineCtrl_PwtrCAN_Rx"
  Bus Selector/1 -> Bus Creator5/1  "<HEVCtrl_Engine_torque_request>"
  Bus Creator5/1 -> Rate Transition1/1
  PwtrCAN/1 -> Bus Selector/1
  [EngineCtrl_PwtrCAN_Tx] -> Unit Delay/1

== system CAN_Lib_V1/Simple_CAN2/Gateway ==
  note: Gateway
  InfoCAN : Inport
  VehCAN : Inport  Port=2
  PwtrCAN : Inport  Port=3
  Gateway_InfoCAN : Subsystem
  Gateway_PwtrCAN : Subsystem
  Gateway_VehCAN : Subsystem
  Info Hub : Subsystem
  Gateway_PwtrCAN_Tx : Outport
  Gateway_VehCAN_Tx : Outport  Port=2
  Gateway_InfoCAN_Tx : Outport  Port=3
  wires:
  Gateway_PwtrCAN/1(Gateway_PwtrCAN_Tx) -> Gateway_PwtrCAN_Tx/1
  Gateway_VehCAN/1(Gateway_VehCAN_Tx) -> Gateway_VehCAN_Tx/1
  Gateway_InfoCAN/1(Gateway_InfoCAN_Tx) -> Gateway_InfoCAN_Tx/1
  VehCAN/1 -> Gateway_PwtrCAN/2(VehCAN), Info Hub/2(VehCAN), Gateway_InfoCAN/1(VehCAN)
  PwtrCAN/1 -> Gateway_VehCAN/2(PwtrCAN), Info Hub/3(PwtrCAN)
  InfoCAN/1 -> Gateway_VehCAN/1(InfoCAN), Gateway_PwtrCAN/1(InfoCAN), Info Hub/1(InfoCAN)

== system CAN_Lib_V1/Simple_CAN2/HEV_Ctrl ==
  note: CAN receive and transmit
  note: HEV control
  note: HEV control
  PwtrCAN : Inport
  Bus Creator1 : BusCreator  Inputs=13
  Bus Selector3 : BusSelector  OutputSignals=BatteryCtrl_PwtrCAN_Tx.BatCtrl_SOC,TransmCtrl_PwtrCAN_Tx.TmCtrl_Clutch_position,TransmCtrl_PwtrCAN_Tx.TmCtrl_Gear_position,Gateway_PwtrCAN_Tx.BrkCtrl_Vehicle_speed,Gateway_PwtrCAN_Tx.BrkCtrl_Regen_brake_torque_request,MotorCtrl_PwtrCAN_Tx.MtrCtrl_Motor_torque_actual,MotorCtrl_PwtrCAN_Tx.MtrCtrl_Motor_torque_available,MotorCtrl_PwtrCAN_Tx.MtrCtrl_Motor_regen_torque_available,EngineCtrl_PwtrCAN_Tx.EngCtrl_Engine_speed,EngineCtrl_PwtrCAN_Tx.EngCtrl_Engine_torque_actual,Gateway_PwtrCAN_Tx.VMCtrl_PropTorqStatus,Gateway_PwtrCAN_Tx.VMCtrl_PropTorqCmnd,Gateway_PwtrCAN_Tx.NAVI_Home_around_status
  Rate Transition1 : RateTransition  Deterministic=off
      settings: AttributesFormatString=<Deterministic=%<Deterministic>>
  Unit Delay : UnitDelay  SampleTime=-1
  HEV_Ctrl_PwtrCAN_Tx : Outport
  tag scope: HEV_Ctrl_PwtrCAN_Rx=scoped
  wires:
  Bus Selector3/13 -> Bus Creator1/13  "<NAVI_Home_around_status>"
  Bus Selector3/12 -> Bus Creator1/12  "<VMCtrl_PropTorqCmnd>"
  Bus Selector3/11 -> Bus Creator1/11  "<VMCtrl_PropTorqStatus>"
  Rate Transition1/1 -> [HEV_Ctrl_PwtrCAN_Rx]  "HEV_Ctrl_PwtrCAN_Rx"
  Unit Delay/1 -> HEV_Ctrl_PwtrCAN_Tx/1  "HEV_Ctrl_PwtrCAN_Tx"
  [HEV_Ctrl_PwtrCAN_Tx] -> Unit Delay/1
  PwtrCAN/1 -> Bus Selector3/1
  Bus Selector3/1 -> Bus Creator1/1  "<BatCtrl_SOC>"
  Bus Selector3/2 -> Bus Creator1/2  "<TmCtrl_Clutch_position>"
  Bus Selector3/3 -> Bus Creator1/3  "<TmCtrl_Gear_position>"
  Bus Selector3/4 -> Bus Creator1/4  "<BrkCtrl_Vehicle_speed>"
  Bus Selector3/5 -> Bus Creator1/5  "<BrkCtrl_Regen_brake_torque_request>"
  Bus Selector3/6 -> Bus Creator1/6  "<MtrCtrl_Motor_torque_actual>"
  Bus Selector3/7 -> Bus Creator1/7  "<MtrCtrl_Motor_torque_available>"
  Bus Selector3/8 -> Bus Creator1/8  "<MtrCtrl_Motor_regen_torque_available>"
  Bus Selector3/9 -> Bus Creator1/9  "<EngCtrl_Engine_speed>"
  Bus Selector3/10 -> Bus Creator1/10  "<EngCtrl_Engine_torque_actual>"
  Bus Creator1/1 -> Rate Transition1/1

== system CAN_Lib_V1/Simple_CAN2/HVAC_Ctrl ==
  note: HVAC Control
  note: CAN receive and transmit
  note: HVAC control
  VehCAN : Inport
  Bus Creator : BusCreator  Inputs=3
  Bus Selector : BusSelector  OutputSignals=Gateway_VehCAN_Tx.EngCtrl_Engine_speed,Gateway_VehCAN_Tx.HEVCtrl_IdleStop_preparation_request,Gateway_VehCAN_Tx.HEVCtrl_IdleStop_status
  Rate Transition1 : RateTransition  Deterministic=off
      settings: AttributesFormatString=<Deterministic=%<Deterministic>>
  Unit Delay : UnitDelay  SampleTime=-1
  HVAC_Ctrl_VehCAN_Tx : Outport
  tag scope: HVAC_Ctrl_VehCAN_Rx=scoped
  wires:
  Bus Selector/3 -> Bus Creator/3  "<HEVCtrl_IdleStop_status>"
  Bus Selector/2 -> Bus Creator/2  "<HEVCtrl_IdleStop_preparation_request>"
  Unit Delay/1 -> HVAC_Ctrl_VehCAN_Tx/1  "HVAC_Ctrl_VehCAN_Tx"
  Rate Transition1/1 -> [HVAC_Ctrl_VehCAN_Rx]  "HVAC_Ctrl_VehCAN_Rx"
  [HVAC_Ctrl_VehCAN_Tx] -> Unit Delay/1
  VehCAN/1 -> Bus Selector/1
  Bus Selector/1 -> Bus Creator/1  "<EngCtrl_Engine_speed>"
  Bus Creator/1 -> Rate Transition1/1

== system CAN_Lib_V1/Simple_CAN2/Motor_Ctrl ==
  note: CAN receive and transmit
  note: Motor Control
  note: Motor control
  PwtrCAN : Inport
  Bus Creator7 : BusCreator  Inputs=3
  Bus Selector2 : BusSelector  OutputSignals=TransmCtrl_PwtrCAN_Tx.TmCtrl_Clutch_position,HEV_Ctrl_PwtrCAN_Tx.HEVCtrl_Motor_torque_request,EngineCtrl_PwtrCAN_Tx.EngCtrl_Engine_speed
  Rate Transition1 : RateTransition  Deterministic=off
      settings: AttributesFormatString=<Deterministic=%<Deterministic>>
  Unit Delay : UnitDelay  SampleTime=-1
  MotorCtrl_PwtrCAN_Tx : Outport
  tag scope: MotorCtrl_PwtrCAN_Rx=scoped
  wires:
  PwtrCAN/1 -> Bus Selector2/1
  Unit Delay/1 -> MotorCtrl_PwtrCAN_Tx/1  "MotorCtrl_PwtrCAN_Tx"
  Bus Selector2/1 -> Bus Creator7/1  "<TmCtrl_Clutch_position>"
  Bus Selector2/3 -> Bus Creator7/3  "<EngCtrl_Engine_speed>"
  Bus Creator7/1 -> Rate Transition1/1
  Bus Selector2/2 -> Bus Creator7/2  "<HEVCtrl_Motor_torque_request>"
  Rate Transition1/1 -> [MotorCtrl_PwtrCAN_Rx]  "MotorCtrl_PwtrCAN_Rx"
  [MotorCtrl_PwtrCAN_Tx] -> Unit Delay/1

== system CAN_Lib_V1/Simple_CAN2/NAVI ==
  note: Navigation
  note: CAN receive and transmit
  note: Navigation
  InfoCAN : Inport
  Bus Creator : BusCreator  Inputs=1
  Bus Selector1 : BusSelector  OutputSignals=Gateway_InfoCAN_Tx.BrkCtrl_Vehicle_speed
  Rate Transition1 : RateTransition  Deterministic=off
      settings: AttributesFormatString=<Deterministic=%<Deterministic>>
  Unit Delay : UnitDelay  SampleTime=-1
  NAVI_InfoCAN_Tx : Outport
  tag scope: NAVI_InfoCAN_Rx=scoped
  wires:
  Unit Delay/1 -> NAVI_InfoCAN_Tx/1  "NAVI_InfoCAN_Tx"
  Rate Transition1/1 -> [NAVI_InfoCAN_Rx]  "NAVI_InfoCAN_Rx"
  [NAVI_InfoCAN_Tx] -> Unit Delay/1
  InfoCAN/1 -> Bus Selector1/1
  Bus Selector1/1 -> Bus Creator/1  "<BrkCtrl_Vehicle_speed>"
  Bus Creator/1 -> Rate Transition1/1

== system CAN_Lib_V1/Simple_CAN2/Radar ==
  note: Radar Detection
  note: CAN receive and transmit
  note: Radar detection
  InfoCAN : Inport
  Bus Creator : BusCreator  Inputs=1
  Bus Selector1 : BusSelector  OutputSignals=Gateway_InfoCAN_Tx.BrkCtrl_Vehicle_speed
  Rate Transition1 : RateTransition  Deterministic=off
      settings: AttributesFormatString=<Deterministic=%<Deterministic>>
  Unit Delay : UnitDelay  SampleTime=-1
  Radar_InfoCAN_Tx : Outport
  tag scope: Radar_InfoCAN_Rx=scoped
  wires:
  Unit Delay/1 -> Radar_InfoCAN_Tx/1  "Radar_InfoCAN_Tx"
  Rate Transition1/1 -> [Radar_InfoCAN_Rx]  "Radar_InfoCAN_Rx"
  [Radar_InfoCAN_Tx] -> Unit Delay/1
  Bus Selector1/1 -> Bus Creator/1  "<BrkCtrl_Vehicle_speed>"
  Bus Creator/1 -> Rate Transition1/1
  InfoCAN/1 -> Bus Selector1/1

== system CAN_Lib_V1/Simple_CAN2/Steer_Ctrl ==
  note: Steering Control
  note: CAN receive and transmit
  note: Steering control
  VehCAN : Inport
  Bus Creator : BusCreator  Inputs=1
  Bus Selector1 : BusSelector  OutputSignals=BrakeCtrl_VehCAN_Tx.BrkCtrl_Vehicle_speed
  Rate Transition1 : RateTransition  Deterministic=off
      settings: AttributesFormatString=<Deterministic=%<Deterministic>>
  Unit Delay : UnitDelay  SampleTime=-1
  SteerCtrl_VehCAN_Tx : Outport
  tag scope: SteerCtrl_VehCAN_Rx=scoped
  wires:
  Unit Delay/1 -> SteerCtrl_VehCAN_Tx/1  "SteerCtrl_VehCAN_Tx"
  Rate Transition1/1 -> [SteerCtrl_VehCAN_Rx]  "SteerCtrl_VehCAN_Rx"
  [SteerCtrl_VehCAN_Tx] -> Unit Delay/1
  VehCAN/1 -> Bus Selector1/1
  Bus Selector1/1 -> Bus Creator/1  "<BrkCtrl_Vehicle_speed>"
  Bus Creator/1 -> Rate Transition1/1

== system CAN_Lib_V1/Simple_CAN2/Transms_Ctrl ==
  note: Transmission Control
  note: CAN receive and transmit
  note: Transmission control
  PwtrCAN : Inport
  Bus Creator6 : BusCreator  Inputs=2
  Bus Selector1 : BusSelector  OutputSignals=Gateway_PwtrCAN_Tx.BrkCtrl_Vehicle_speed,EngineCtrl_PwtrCAN_Tx.EngCtrl_Engine_speed
  Rate Transition1 : RateTransition  Deterministic=off
      settings: AttributesFormatString=<Deterministic=%<Deterministic>>
  Unit Delay : UnitDelay  SampleTime=-1
  TransmCtrl_PwtrCAN_Tx : Outport
  tag scope: TransmCtrl_PwtrCAN_Rx=scoped
  wires:
  Rate Transition1/1 -> [TransmCtrl_PwtrCAN_Rx]  "TransmCtrl_PwtrCAN_Rx"
  PwtrCAN/1 -> Bus Selector1/1
  Bus Selector1/1 -> Bus Creator6/1  "<BrkCtrl_Vehicle_speed>"
  Bus Selector1/2 -> Bus Creator6/2  "<EngCtrl_Engine_speed>"
  Bus Creator6/1 -> Rate Transition1/1
  Unit Delay/1 -> TransmCtrl_PwtrCAN_Tx/1  "TransmCtrl_PwtrCAN_Tx"
  [TransmCtrl_PwtrCAN_Tx] -> Unit Delay/1

== system CAN_Lib_V1/Simple_CAN2/VM_Ctrl ==
  note: CAN receive and transmit
  note: Vehicle Motion Control
  note: Vehicle motion control
  VehCAN : Inport
  Bus Creator : BusCreator  Inputs=1
  Bus Selector1 : BusSelector  OutputSignals=BrakeCtrl_VehCAN_Tx.BrkCtrl_Vehicle_speed
  Rate Transition1 : RateTransition  Deterministic=off
      settings: AttributesFormatString=<Deterministic=%<Deterministic>>
  Unit Delay : UnitDelay  SampleTime=-1
  VM_Ctrl_VehCAN_Tx : Outport
  tag scope: VM_Ctrl_VehCAN_Rx=scoped
  wires:
  Unit Delay/1 -> VM_Ctrl_VehCAN_Tx/1  "VM_Ctrl_VehCAN_Tx"
  Rate Transition1/1 -> [VM_Ctrl_VehCAN_Rx]  "VM_Ctrl_VehCAN_Rx"
  [VM_Ctrl_VehCAN_Tx] -> Unit Delay/1
  VehCAN/1 -> Bus Selector1/1
  Bus Selector1/1 -> Bus Creator/1  "<BrkCtrl_Vehicle_speed>"
  Bus Creator/1 -> Rate Transition1/1

== system CAN_Lib_V1/Simple_CAN_Integ/Battery_Ctrl ==
  note: Battery Control
  note: CAN receive and transmit
  note: Battery control
  CAN : Inport
  Rate Transition1 : RateTransition  Deterministic=off
      settings: AttributesFormatString=<Deterministic=%<Deterministic>>
  Rate Transition2 : RateTransition  Deterministic=off
      settings: AttributesFormatString=<Deterministic=%<Deterministic>>
  BatteryCtrl_PwtrCAN_Tx : Outport
  tag scope: BatteryCtrl_PwtrCAN_Rx=scoped
  wires:
  CAN/1 -> Rate Transition1/1
  Rate Transition2/1 -> BatteryCtrl_PwtrCAN_Tx/1  "BatteryCtrl_PwtrCAN_Tx"
  Rate Transition1/1 -> [BatteryCtrl_PwtrCAN_Rx]  "BatteryCtrl_PwtrCAN_Rx"
  [BatteryCtrl_PwtrCAN_Tx] -> Rate Transition2/1

== system CAN_Lib_V1/Simple_CAN_Integ/Body_Ctrl ==
  note: Body Control
  note: CAN receive and transmit
  note: Body control
  CAN : Inport
  Rate Transition1 : RateTransition  Deterministic=off
      settings: AttributesFormatString=<Deterministic=%<Deterministic>>
  Rate Transition2 : RateTransition  Deterministic=off
      settings: AttributesFormatString=<Deterministic=%<Deterministic>>
  BodyCtrl_VehCAN_Tx : Outport
  tag scope: BodyCtrl_VehCAN_Rx=scoped
  wires:
  CAN/1 -> Rate Transition1/1
  Rate Transition2/1 -> BodyCtrl_VehCAN_Tx/1  "BodyCtrl_VehCAN_Tx"
  Rate Transition1/1 -> [BodyCtrl_VehCAN_Rx]  "BodyCtrl_VehCAN_Rx"
  [BodyCtrl_VehCAN_Tx] -> Rate Transition2/1

== system CAN_Lib_V1/Simple_CAN_Integ/Brake_Ctrl ==
  note: Brake Control
  note: CAN receive and transmit
  note: Brake control
  CAN : Inport
  Rate Transition1 : RateTransition  Deterministic=off
      settings: AttributesFormatString=<Deterministic=%<Deterministic>>
  Rate Transition2 : RateTransition  Deterministic=off
      settings: AttributesFormatString=<Deterministic=%<Deterministic>>
  BrakeCtrl_VehCAN_Tx : Outport
  tag scope: BrakeCtrl_VehCAN_Rx=scoped
  wires:
  CAN/1 -> Rate Transition1/1
  Rate Transition2/1 -> BrakeCtrl_VehCAN_Tx/1  "BrakeCtrl_VehCAN_Tx"
  Rate Transition1/1 -> [BrakeCtrl_VehCAN_Rx]  "BrakeCtrl_VehCAN_Rx"
  [BrakeCtrl_VehCAN_Tx] -> Rate Transition2/1

== system CAN_Lib_V1/Simple_CAN_Integ/Engine_Ctrl ==
  note: CAN receive and transmit
  note: Engine Control
  note: Engine control
  CAN : Inport
  Rate Transition1 : RateTransition  Deterministic=off
      settings: AttributesFormatString=<Deterministic=%<Deterministic>>
  Rate Transition2 : RateTransition  Deterministic=off
      settings: AttributesFormatString=<Deterministic=%<Deterministic>>
  EngineCtrl_PwtrCAN_Tx : Outport
  tag scope: EngineCtrl_PwtrCAN_Rx=scoped
  wires:
  Rate Transition2/1 -> EngineCtrl_PwtrCAN_Tx/1  "EngineCtrl_PwtrCAN_Tx"
  Rate Transition1/1 -> [EngineCtrl_PwtrCAN_Rx]  "EngineCtrl_PwtrCAN_Rx"
  CAN/1 -> Rate Transition1/1
  [EngineCtrl_PwtrCAN_Tx] -> Rate Transition2/1

== system CAN_Lib_V1/Simple_CAN_Integ/HEV_Ctrl ==
  note: CAN receive and transmit
  note: HEV control
  note: HEV control
  CAN : Inport
  Rate Transition1 : RateTransition  Deterministic=off
      settings: AttributesFormatString=<Deterministic=%<Deterministic>>
  Rate Transition4 : RateTransition  Deterministic=off
      settings: AttributesFormatString=<Deterministic=%<Deterministic>>
  HEV_Ctrl_PwtrCAN_Tx : Outport
  tag scope: HEV_Ctrl_PwtrCAN_Rx=scoped
  wires:
  Rate Transition1/1 -> [HEV_Ctrl_PwtrCAN_Rx]  "HEV_Ctrl_PwtrCAN_Rx"
  Rate Transition4/1 -> HEV_Ctrl_PwtrCAN_Tx/1  "HEV_Ctrl_PwtrCAN_Tx"
  [HEV_Ctrl_PwtrCAN_Tx] -> Rate Transition4/1
  CAN/1 -> Rate Transition1/1

== system CAN_Lib_V1/Simple_CAN_Integ/HVAC_Ctrl ==
  note: HVAC Control
  note: CAN receive and transmit
  note: HVAC control
  CAN : Inport
  Rate Transition1 : RateTransition  Deterministic=off
      settings: AttributesFormatString=<Deterministic=%<Deterministic>>
  Rate Transition2 : RateTransition  Deterministic=off
      settings: AttributesFormatString=<Deterministic=%<Deterministic>>
  HVAC_Ctrl_VehCAN_Tx : Outport
  tag scope: HVAC_Ctrl_VehCAN_Rx=scoped
  wires:
  Rate Transition2/1 -> HVAC_Ctrl_VehCAN_Tx/1  "HVAC_Ctrl_VehCAN_Tx"
  Rate Transition1/1 -> [HVAC_Ctrl_VehCAN_Rx]  "HVAC_Ctrl_VehCAN_Rx"
  [HVAC_Ctrl_VehCAN_Tx] -> Rate Transition2/1
  CAN/1 -> Rate Transition1/1

== system CAN_Lib_V1/Simple_CAN_Integ/Motor_Ctrl ==
  note: CAN receive and transmit
  note: Motor Control
  note: Motor control
  CAN : Inport
  Rate Transition1 : RateTransition  Deterministic=off
      settings: AttributesFormatString=<Deterministic=%<Deterministic>>
  Rate Transition2 : RateTransition  Deterministic=off
      settings: AttributesFormatString=<Deterministic=%<Deterministic>>
  MotorCtrl_PwtrCAN_Tx : Outport
  tag scope: MotorCtrl_PwtrCAN_Rx=scoped
  wires:
  Rate Transition2/1 -> MotorCtrl_PwtrCAN_Tx/1  "MotorCtrl_PwtrCAN_Tx"
  CAN/1 -> Rate Transition1/1
  Rate Transition1/1 -> [MotorCtrl_PwtrCAN_Rx]  "MotorCtrl_PwtrCAN_Rx"
  [MotorCtrl_PwtrCAN_Tx] -> Rate Transition2/1

== system CAN_Lib_V1/Simple_CAN_Integ/NAVI ==
  note: Navigation
  note: CAN receive and transmit
  note: Navigation
  CAN : Inport
  Rate Transition1 : RateTransition  Deterministic=off
      settings: AttributesFormatString=<Deterministic=%<Deterministic>>
  Rate Transition2 : RateTransition  Deterministic=off
      settings: AttributesFormatString=<Deterministic=%<Deterministic>>
  NAVI_InfoCAN_Tx : Outport
  tag scope: NAVI_InfoCAN_Rx=scoped
  wires:
  Rate Transition2/1 -> NAVI_InfoCAN_Tx/1  "NAVI_InfoCAN_Tx"
  Rate Transition1/1 -> [NAVI_InfoCAN_Rx]  "NAVI_InfoCAN_Rx"
  [NAVI_InfoCAN_Tx] -> Rate Transition2/1
  CAN/1 -> Rate Transition1/1

== system CAN_Lib_V1/Simple_CAN_Integ/Radar ==
  note: Radar Detection
  note: CAN receive and transmit
  note: Radar detection
  CAN : Inport
  Rate Transition1 : RateTransition  Deterministic=off
      settings: AttributesFormatString=<Deterministic=%<Deterministic>>
  Rate Transition2 : RateTransition  Deterministic=off
      settings: AttributesFormatString=<Deterministic=%<Deterministic>>
  Radar_InfoCAN_Tx : Outport
  tag scope: Radar_InfoCAN_Rx=scoped
  wires:
  Rate Transition2/1 -> Radar_InfoCAN_Tx/1  "Radar_InfoCAN_Tx"
  Rate Transition1/1 -> [Radar_InfoCAN_Rx]  "Radar_InfoCAN_Rx"
  [Radar_InfoCAN_Tx] -> Rate Transition2/1
  CAN/1 -> Rate Transition1/1

== system CAN_Lib_V1/Simple_CAN_Integ/Steer_Ctrl ==
  note: Steering Control
  note: CAN receive and transmit
  note: Steering control
  CAN : Inport
  Rate Transition1 : RateTransition  Deterministic=off
      settings: AttributesFormatString=<Deterministic=%<Deterministic>>
  Rate Transition2 : RateTransition  Deterministic=off
      settings: AttributesFormatString=<Deterministic=%<Deterministic>>
  SteerCtrl_VehCAN_Tx : Outport
  tag scope: SteerCtrl_VehCAN_Rx=scoped
  wires:
  CAN/1 -> Rate Transition1/1
  Rate Transition2/1 -> SteerCtrl_VehCAN_Tx/1  "SteerCtrl_VehCAN_Tx"
  Rate Transition1/1 -> [SteerCtrl_VehCAN_Rx]  "SteerCtrl_VehCAN_Rx"
  [SteerCtrl_VehCAN_Tx] -> Rate Transition2/1

== system CAN_Lib_V1/Simple_CAN_Integ/Transms_Ctrl ==
  note: Transmission Control
  note: CAN receive and transmit
  note: Transmission control
  CAN : Inport
  Rate Transition1 : RateTransition  Deterministic=off
      settings: AttributesFormatString=<Deterministic=%<Deterministic>>
  Rate Transition2 : RateTransition  Deterministic=off
      settings: AttributesFormatString=<Deterministic=%<Deterministic>>
  TransmCtrl_PwtrCAN_Tx : Outport
  tag scope: TransmCtrl_PwtrCAN_Rx=scoped
  wires:
  Rate Transition1/1 -> [TransmCtrl_PwtrCAN_Rx]  "TransmCtrl_PwtrCAN_Rx"
  CAN/1 -> Rate Transition1/1
  Rate Transition2/1 -> TransmCtrl_PwtrCAN_Tx/1  "TransmCtrl_PwtrCAN_Tx"
  [TransmCtrl_PwtrCAN_Tx] -> Rate Transition2/1
